simulink model "tractor_trailer_system"  (R2021a)
settings: Solver=VariableStepAuto  StartTime=0.0  StopTime=10.0  RelTol=1e-3
values from neighbouring files (symbols this model uses):
  lr1 = 2.9    [linear_lqr.m]    (also in linear_mpc.m)
  lt1 = 1.8    [linear_lqr.m]    (also in linear_mpc.m)
  m0 = 0.8    [linear_lqr.m]    (also in linear_mpc.m)
  tau = 0.3    [linear_lqr.m]    (also in linear_mpc.m)
settings Model: Creator=haquo  LastModifiedBy=haquo

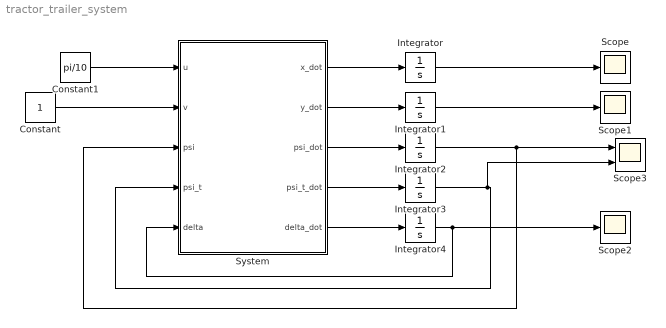
== system tractor_trailer_system ==
  Constant : Constant
  Constant1 : Constant  Value=pi/10
  Integrator : Integrator
  Integrator1 : Integrator
  Integrator2 : Integrator
  Integrator3 : Integrator  InitialCondition=pi/8
  Integrator4 : Integrator  InitialCondition=0.0
  Scope : Scope
  Scope1 : Scope
  Scope2 : Scope
  Scope3 : Scope  NumInputPorts=2
  System : MATLAB Function  TreatAsAtomicUnit=on
  wires:
  System/5(delta_dot) -> Integrator4/1
  System/4(psi_t_dot) -> Integrator3/1
  System/3(psi_dot) -> Integrator2/1
  System/2(y_dot) -> Integrator1/1
  System/1(x_dot) -> Integrator/1
  Integrator2/1 -> Scope3/1, System/3(psi)
  Integrator/1 -> Scope/1
  Integrator1/1 -> Scope1/1
  Integrator4/1 -> System/5(delta), Scope2/1
  Constant/1 -> System/2(v)
  Constant1/1 -> System/1(u)
  Integrator3/1 -> Scope3/2, System/4(psi_t)

== matlab function tractor_trailer_system/System ==
  data: u input; x_dot output; v input; psi input; psi_t input; delta input; y_dot output; psi_dot output; psi_t_dot output; delta_dot output; m0 parameter; tau parameter; lt1 parameter; lr1 parameter
function [x_dot, y_dot, psi_dot, psi_t_dot, delta_dot] = fcn(u, v, psi, psi_t, delta, m0, tau, lt1, lr1)

x_dot = v * cos(psi);
y_dot = v * sin(psi);
psi_dot = v * tan(delta) / lr1;
psi_t_dot = (v / lt1) * sin(psi - psi_t) - (m0*v / lr1*lt1) * cos(psi - psi_t) * tan(delta);
delta_dot = - (1/tau) * (delta - u);

end
